simulink subsystem "getAccelDataNew"  (R2024a)
settings: Solver=VariableStepAuto  StartTime=0.0  StopTime=10.0  RelTol=1e-3
undefined symbols (not defined in the file or in its folder): bits, measRate
libraries: stm32blockslib x7
settings Model: Creator=Peter  LastModifiedBy=Peter

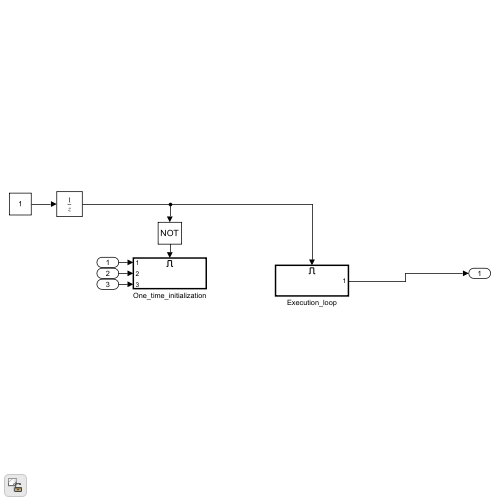
[thumbnail: Simulink's stored preview of the top-level diagram]
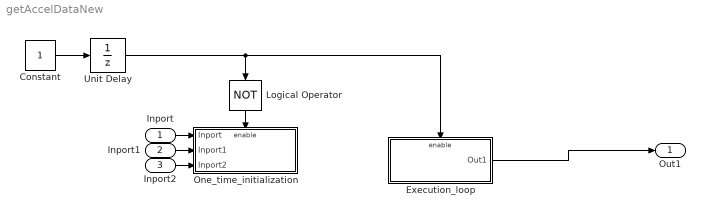
== system getAccelDataNew ==
  Inport : Inport
  Inport1 : Inport  Port=2
  Inport2 : Inport  Port=3
  Constant : Constant  OutDataTypeStr=boolean  SampleTime=measRate
  Execution_loop : Subsystem  TreatAsAtomicUnit=on
  Logical Operator : Logic  Operator=NOT  AllPortsSameDT=off  OutDataTypeStr=boolean
  One_time_initialization : Subsystem  TreatAsAtomicUnit=on
  Unit Delay : UnitDelay  SampleTime=-1  HasFrameUpgradeWarning=on
  Out1 : Outport
  wires:
  Execution_loop/1(Out1) -> Out1/1
  Unit Delay/1 -> Logical Operator/1, Execution_loop/Enable
  Constant/1 -> Unit Delay/1
  Inport1/1 -> One_time_initialization/2(Inport1)
  Logical Operator/1 -> One_time_initialization/Enable
  Inport/1 -> One_time_initialization/1(Inport)
  Inport2/1 -> One_time_initialization/3(Inport2)

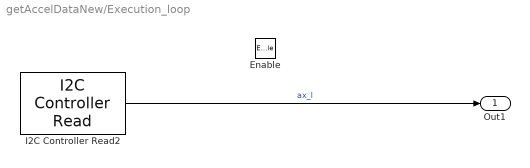
== system getAccelDataNew/Execution_loop ==
  Enable : EnablePort
  I2C Controller Read2 : stm32blockslib/I2C Controller Read  Priority=-1  I2CModule=I2C2  Mode=Controller  AddressingMode=7-bits  PeripheralByteOrder=LittleEndian  OwnPeripheralAddress=uint8(170)  PeripheralAddressVia=Dialog  PeripheralAddress=hex2dec('53')  RegisterAddressMode=on  RegisterAddressVia=Dialog  RegisterAddress=uint8(hex2dec('32'))  RepeatedStart=off  NoAck=off  OutputStatus=off  BlockMode=Receive  DataType=uint8  DataLength=6  Timeout=0.001  SampleTime=inf
      settings: LibrarySourceBlock=stm32f7xxblockslib/I2C Controller Read
  Out1 : Outport  VectorParamsAs1DForOutWhenUnconnected=off
  wires:
  I2C Controller Read2/1 -> Out1/1  "ax_l"

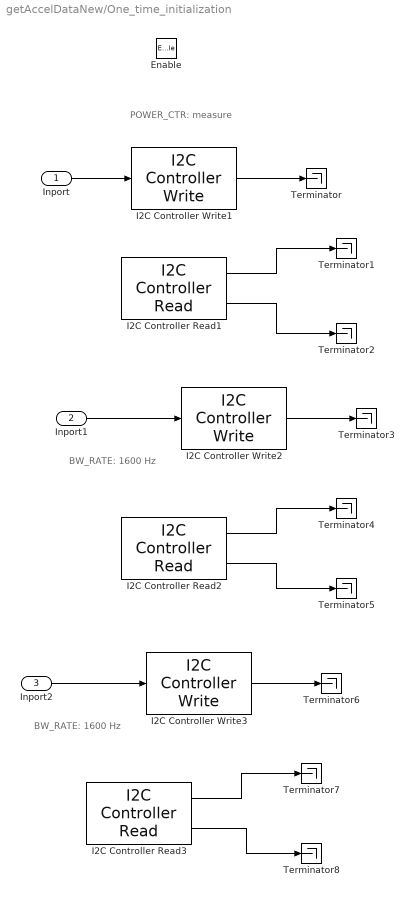
== system getAccelDataNew/One_time_initialization ==
  note: BW_RATE: 1600 Hz
  note: BW_RATE: 1600 Hz
  note: POWER_CTR: measure
  Inport : Inport
  Inport1 : Inport  Port=2
  Inport2 : Inport  Port=3
  Enable : EnablePort
  I2C Controller Read1 : stm32blockslib/I2C Controller Read  Priority=-4  I2CModule=I2C2  Mode=Controller  AddressingMode=7-bits  PeripheralByteOrder=LittleEndian  OwnPeripheralAddress=uint8(170)  PeripheralAddressVia=Dialog  PeripheralAddress=hex2dec('53')  RegisterAddressMode=on  RegisterAddressVia=Dialog  RegisterAddress=uint8(hex2dec('2D'))  RepeatedStart=off  NoAck=off  OutputStatus=on  BlockMode=Receive  DataType=uint8  DataLength=1  Timeout=0.001  SampleTime=inf
      settings: LibrarySourceBlock=stm32f7xxblockslib/I2C Controller Read
  I2C Controller Read2 : stm32blockslib/I2C Controller Read  Priority=-2  I2CModule=I2C2  Mode=Controller  AddressingMode=7-bits  PeripheralByteOrder=LittleEndian  OwnPeripheralAddress=uint8(170)  PeripheralAddressVia=Dialog  PeripheralAddress=hex2dec('53')  RegisterAddressMode=on  RegisterAddressVia=Dialog  RegisterAddress=uint8(hex2dec('2C'))  RepeatedStart=off  NoAck=off  OutputStatus=on  BlockMode=Receive  DataType=uint8  DataLength=1  Timeout=0.001  SampleTime=inf
      settings: LibrarySourceBlock=stm32f7xxblockslib/I2C Controller Read
  I2C Controller Read3 : stm32blockslib/I2C Controller Read  Priority=-2  I2CModule=I2C2  Mode=Controller  AddressingMode=7-bits  PeripheralByteOrder=LittleEndian  OwnPeripheralAddress=uint8(170)  PeripheralAddressVia=Dialog  PeripheralAddress=hex2dec('53')  RegisterAddressMode=on  RegisterAddressVia=Dialog  RegisterAddress=uint8(hex2dec('2C'))  RepeatedStart=off  NoAck=off  OutputStatus=on  BlockMode=Receive  DataType=uint8  DataLength=1  Timeout=0.001  SampleTime=inf
      settings: LibrarySourceBlock=stm32f7xxblockslib/I2C Controller Read
  I2C Controller Write1 : stm32blockslib/I2C Controller Write  Priority=-5  I2CModule=I2C2  Mode=Controller  AddressingMode=7-bits  PeripheralByteOrder=LittleEndian  OwnPeripheralAddress=uint8(170)  PeripheralAddressVia=Dialog  PeripheralAddress=hex2dec('53')  RegisterAddressMode=on  RegisterAddressVia=Dialog  RegisterAddress=uint8(hex2dec('2D'))  RepeatedStart=off  NoAck=off  OutputStatus=on  BlockMode=Transmit  DataType=uint8  DataLength=1  Timeout=0.001  SampleTime=-1
      settings: LibrarySourceBlock=stm32f7xxblockslib/I2C Controller Write
  I2C Controller Write2 : stm32blockslib/I2C Controller Write  Priority=-3  I2CModule=I2C2  Mode=Controller  AddressingMode=7-bits  PeripheralByteOrder=LittleEndian  OwnPeripheralAddress=uint8(170)  PeripheralAddressVia=Dialog  PeripheralAddress=hex2dec('53')  RegisterAddressMode=on  RegisterAddressVia=Dialog  RegisterAddress=uint8(hex2dec('2C'))  RepeatedStart=off  NoAck=off  OutputStatus=on  BlockMode=Transmit  DataType=uint8  DataLength=1  Timeout=0.001  SampleTime=-1
      settings: LibrarySourceBlock=stm32f7xxblockslib/I2C Controller Write
  I2C Controller Write3 : stm32blockslib/I2C Controller Write  Priority=-3  I2CModule=I2C2  Mode=Controller  AddressingMode=7-bits  PeripheralByteOrder=LittleEndian  OwnPeripheralAddress=uint8(170)  PeripheralAddressVia=Dialog  PeripheralAddress=hex2dec('53')  RegisterAddressMode=on  RegisterAddressVia=Dialog  RegisterAddress=uint8(hex2dec('31'))  RepeatedStart=off  NoAck=off  OutputStatus=on  BlockMode=Transmit  DataType=uint8  DataLength=1  Timeout=0.001  SampleTime=-1
      settings: LibrarySourceBlock=stm32f7xxblockslib/I2C Controller Write
  Terminator{,1..8} (9 alike) : Terminator
  wires:
  I2C Controller Read3/1 -> Terminator7/1
  I2C Controller Write3/1 -> Terminator6/1
  Inport2/1 -> I2C Controller Write3/1
  I2C Controller Read3/2 -> Terminator8/1
  I2C Controller Read2/2 -> Terminator5/1
  Inport1/1 -> I2C Controller Write2/1
  I2C Controller Write2/1 -> Terminator3/1
  Inport/1 -> I2C Controller Write1/1
  I2C Controller Read2/1 -> Terminator4/1
  I2C Controller Read1/2 -> Terminator2/1
  I2C Controller Read1/1 -> Terminator1/1
  I2C Controller Write1/1 -> Terminator/1
